simulink model "subsystem_discrete"  (R2015a)
settings: Solver=ode45  StartTime=0.0  StopTime=20  RelTol=1e-3
undefined symbols (not defined in the file): F, F_delay, J, K, Ki, Kp, R, ref
settings Model: Creator=Max  LastModifiedBy=Max

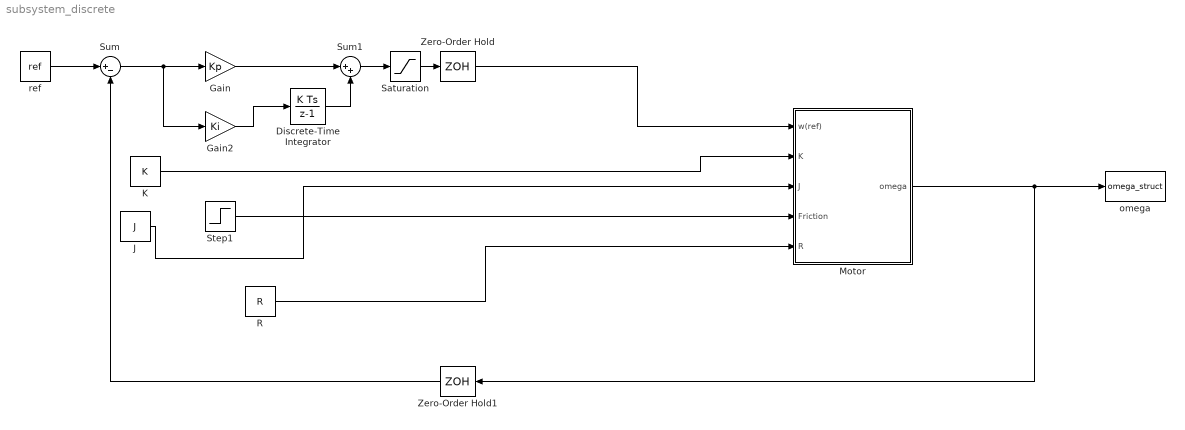
== system subsystem_discrete ==
  Discrete-Time Integrator : DiscreteIntegrator  InitialConditionSetting=State (most efficient)
  Gain : Gain  Gain=Kp
  Gain2 : Gain  Gain=Ki
  J : Constant  Value=J
  K : Constant  Value=K
  Motor : Subsystem
  R : Constant  Value=R
  Saturation : Saturate  UpperLimit=6  LowerLimit=-6
  Step1 : Step  Time=F_delay  After=F  SampleTime=0
  Sum : Sum  Inputs=|+-
  Sum1 : Sum  Inputs=|++
  Zero-Order Hold : ZeroOrderHold
  Zero-Order Hold1 : ZeroOrderHold
  omega : ToWorkspace  VariableName=omega_struct  SaveFormat=Structure With Time  SampleTime=-1
  ref : Constant  Value=ref
  wires:
  ref/1 -> Sum/1
  Sum/1 -> Gain2/1, Gain/1
  Gain2/1 -> Discrete-Time Integrator/1
  Discrete-Time Integrator/1 -> Sum1/2
  Motor/1(omega) -> Zero-Order Hold1/1, omega/1
  Step1/1 -> Motor/4(Friction)
  K/1 -> Motor/2(K)
  R/1 -> Motor/5(R)
  J/1 -> Motor/3(J)
  Gain/1 -> Sum1/1
  Zero-Order Hold1/1 -> Sum/2
  Saturation/1 -> Zero-Order Hold/1
  Sum1/1 -> Saturation/1
  Zero-Order Hold/1 -> Motor/1(w(ref))

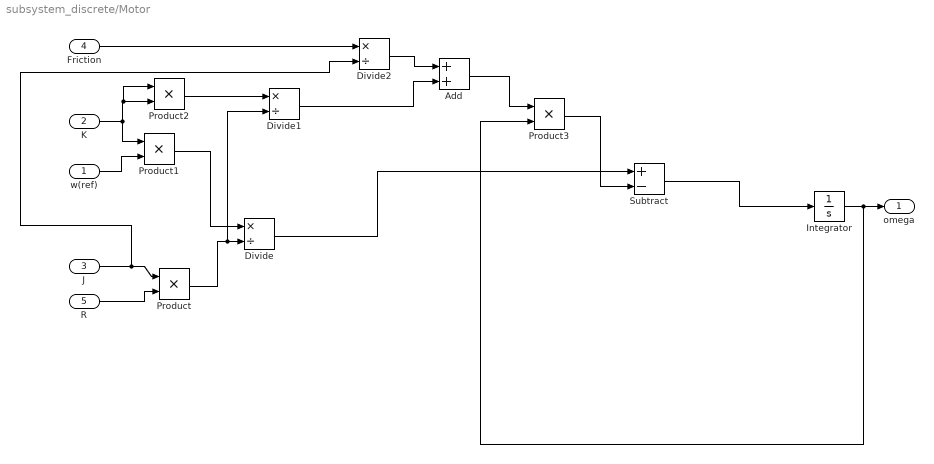
== system subsystem_discrete/Motor ==
  w(ref) : Inport
  K : Inport  Port=2
  J : Inport  Port=3
  Friction : Inport  Port=4
  R : Inport  Port=5
  Add : Sum
  Divide : Product  Inputs=*/
  Divide1 : Product  Inputs=*/
  Divide2 : Product  Inputs=*/
  Integrator : Integrator
  Product{,1..3} (4 alike) : Product
  Subtract : Sum  Inputs=+-
  omega : Outport
  wires:
  R/1 -> Product/2
  Product/1 -> Divide1/2, Divide/2
  K/1 -> Product1/1, Product2/1, Product2/2
  w(ref)/1 -> Product1/2
  Product1/1 -> Divide/1
  Product2/1 -> Divide1/1
  Friction/1 -> Divide2/1
  J/1 -> Divide2/2, Product/1
  Divide2/1 -> Add/1
  Divide1/1 -> Add/2
  Add/1 -> Product3/1
  Integrator/1 -> Product3/2, omega/1
  Product3/1 -> Subtract/2
  Divide/1 -> Subtract/1
  Subtract/1 -> Integrator/1
